simulink model "E2"  (R2023a)
settings: Solver=VariableStepAuto  StartTime=0.0  StopTime=0.08  MaxStep=1e-4  RelTol=1e-3
settings Model: Creator=swara  LastModifiedBy=swara

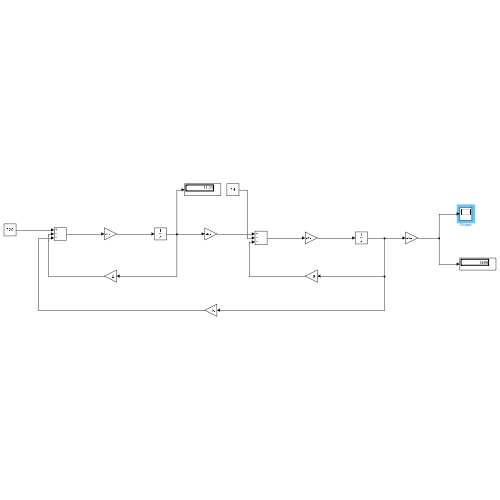
[thumbnail: Simulink's stored preview of the top-level diagram]
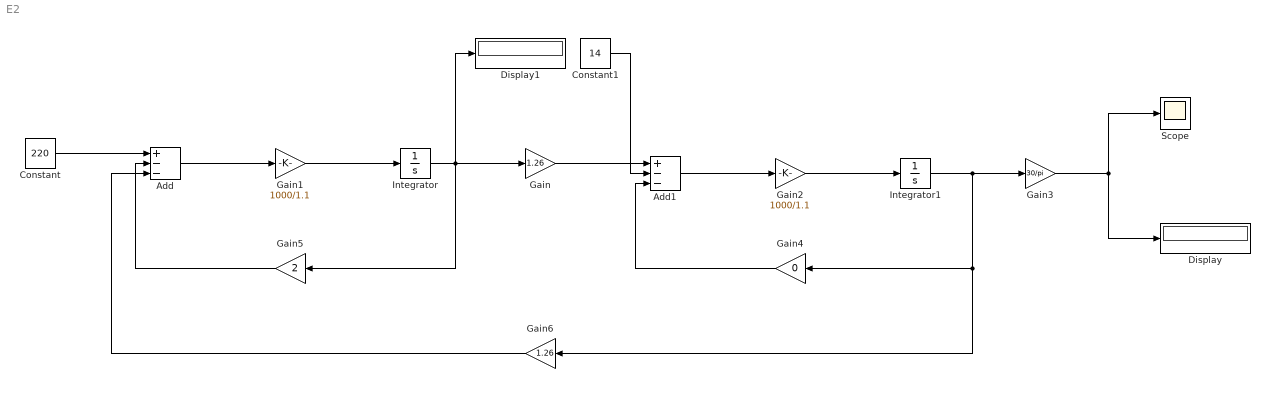
== system E2 ==
  Add : Sum  Inputs=+--
  Add1 : Sum  Inputs=+--
  Constant : Constant  Value=220
  Constant1 : Constant  Value=14
  Display : Display
  Display1 : Display
  Gain : Gain  Gain=1.26
  Gain1 : Gain  Gain=1000/1.1
  Gain2 : Gain  Gain=1000/1.1
  Gain3 : Gain  Gain=30/pi
  Gain4 : Gain  Gain=0
  Gain5 : Gain  Gain=2
  Gain6 : Gain  Gain=1.26
  Integrator : Integrator
  Integrator1 : Integrator
  Scope : Scope
  wires:
  Constant/1 -> Add/1
  Add/1 -> Gain1/1
  Gain1/1 -> Integrator/1
  Integrator/1 -> Gain5/1, Gain/1, Display1/1
  Gain3/1 -> Scope/1, Display/1
  Integrator1/1 -> Gain4/1, Gain6/1, Gain3/1
  Gain2/1 -> Integrator1/1
  Add1/1 -> Gain2/1
  Gain/1 -> Add1/1
  Constant1/1 -> Add1/2
  Gain5/1 -> Add/2
  Gain6/1 -> Add/3
  Gain4/1 -> Add1/3
